simulink model "Sim"  (R2018a)
settings: Solver=VariableStepAuto  StartTime=0.0  StopTime=20  RelTol=1e-3
values from neighbouring files (symbols this model uses):
  A = [ 0 0 1 0 0 ; 0 0 0 1 0 ; -(k1+k2)/m1 k2/m1 0 0 1/m1 ; k2/m2 -k2/m2 0 0 0 ; 0 0 0 0 0]    [Example_Simulink.m]    (also in Example_matlab.m)
  B = [0;0;0;0;1]    [Example_Simulink.m]    (also in Example_matlab.m)
  K = place(A,B,Poles)    [Example_Simulink.m]    (also in Example_matlab.m)
  N = numel(t)    [Example_Simulink.m]    (also in Example_matlab.m)
  r = 10    [Example_Simulink.m]    (also in Example_matlab.m)
settings Model: Creator=Sorawit Inprom  LastModifiedBy=Sorawit Inprom

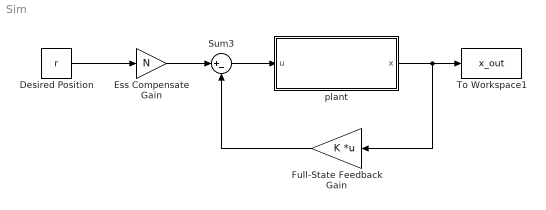
== system Sim ==
  Desired Position : Constant  Value=r
  Ess Compensate Gain : Gain  Gain=N
  Full-State Feedback Gain : Gain  Gain=K  Multiplication=Matrix(K*u)
  Sum3 : Sum  Inputs=|+-
  To Workspace1 : ToWorkspace  VariableName=x_out  SaveFormat=Timeseries  SampleTime=-1
  plant : Subsystem
  wires:
  Ess Compensate Gain/1 -> Sum3/1
  Desired Position/1 -> Ess Compensate Gain/1
  Full-State Feedback Gain/1 -> Sum3/2
  plant/1(x) -> Full-State Feedback Gain/1, To Workspace1/1
  Sum3/1 -> plant/1(u)

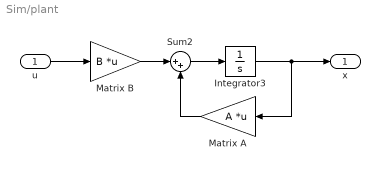
== system Sim/plant ==
  u : Inport
  Integrator3 : Integrator  InitialCondition=[0 0 0 0 0 ]
  Matrix A : Gain  Gain=A  Multiplication=Matrix(K*u)
  Matrix B : Gain  Gain=B  Multiplication=Matrix(K*u)
  Sum2 : Sum  Inputs=|++
  x : Outport
  wires:
  Sum2/1 -> Integrator3/1
  Integrator3/1 -> x/1, Matrix A/1
  Matrix A/1 -> Sum2/2
  Matrix B/1 -> Sum2/1
  u/1 -> Matrix B/1
